simulink model "V30x2810x29"  (R2024b)
settings: Solver=ode1  StartTime=0.0  StopTime=inf  FixedStep=0.01  RelTol=1e-3  EnableMultiTasking=on
PostLoadFcn:
  | qlabs_setup
model workspace (MAT data in the model file):
  Sig = Simulink.Signal
  Sig.Dimensions = -1
  Sig.DimensionsMode = 'auto'
  Sig.Complexity = 'auto'
  Sig.SampleTime = -1
  Sig.SamplingMode = 'auto'
  Sig.DataType = 'auto'
  downCamStepSize = Simulink.Parameter
  downCamStepSize.Value = Simulink.data.Expression
  downCamStepSize.Value.ExpressionString = "qc_get_step_size*ceil(1/30/qc_get_step_size)"
  downCamStepSize.Complexity = 'real'
  downCamStepSize.Dimensions = -1
  downCamStepSize.DataType = 'auto'
  lidarStepSize = Simulink.Parameter
  lidarStepSize.Value = Simulink.data.Expression
  lidarStepSize.Value.ExpressionString = "qc_get_step_size*ceil(1/5/qc_get_step_size)"
  lidarStepSize.Complexity = 'real'
  lidarStepSize.Dimensions = -1
  lidarStepSize.DataType = 'auto'
  mainStepSize = Simulink.Parameter
  mainStepSize.Value = Simulink.data.Expression
  mainStepSize.Value.ExpressionString = "qc_get_step_size"
  mainStepSize.Complexity = 'real'
  mainStepSize.Dimensions = -1
  mainStepSize.DataType = 'auto'
  mode = Simulink.Parameter
  mode.Value = 2
  mode.Complexity = 'real'
  mode.Dimensions = [1 1]
  mode.Description = '0 - education speeds via wheel speed commands
    | 1 - education speeds via body speed commands
    | 2 - research speeds via wheel speed commands
    | 3 - research speeds via body speed commands'
  mode.DataType = 'auto'
  realSenseStepSize = Simulink.Parameter
  realSenseStepSize.Value = Simulink.data.Expression
  realSenseStepSize.Value.ExpressionString = "qc_get_step_size*ceil(1/30/qc_get_step_size)"
  realSenseStepSize.Complexity = 'real'
  realSenseStepSize.Dimensions = -1
  realSenseStepSize.DataType = 'auto'
values from neighbouring files (symbols this model uses):
  obstacles = [ ... (first row only)    [init.m]
  waypoints = [ ... (first row only)    [init.m]
libraries: quarc_library x7
settings Model: ExtModeTrigDuration=10000  Creator=mbohra  LastModifiedBy=simon
settings SolverCC: PositivePriorityOrder=on
settings DebuggingCC: UnderspecifiedInitializationDetection=Classic  MergeDetectMultiDrivingBlocksExec=none
settings ModelReferenceCC: PropagateSignalLabelsOutOfModel=off
settings RTWCC: Description=QUARC Win64 Target Using Toolchain  SystemTargetFile=quarc_win64.tlc  Toolchain=QUARC win64 | nmake (64-bit Windows)  BuildConfiguration=Faster Runs  GPUComputeCapability=3.5
settings STFCustomTargetCC: TargetLangStandard=C99 (ISO)  ConcurrentExecutionCompliant=on  GRTInterface=on  UseToolchainInfoCompliant=on  SystemTargetFile=quarc_win64.tlc
settings GRTTargetCC: ParMdlRefBuildCompliant=off  CompOptLevelCompliant=off  CombineOutputUpdateFcns=off  MatFileLogging=off  CPPClassGenCompliant=off  GRTInterface=on  ExtMode=on  ExtModeMexFile=quarc_comm

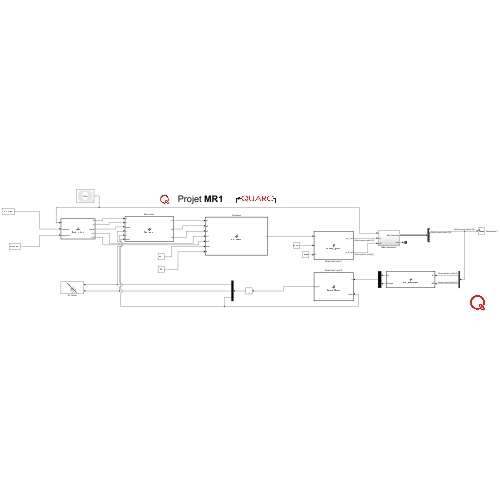
[thumbnail: Simulink's stored preview of the top-level diagram]
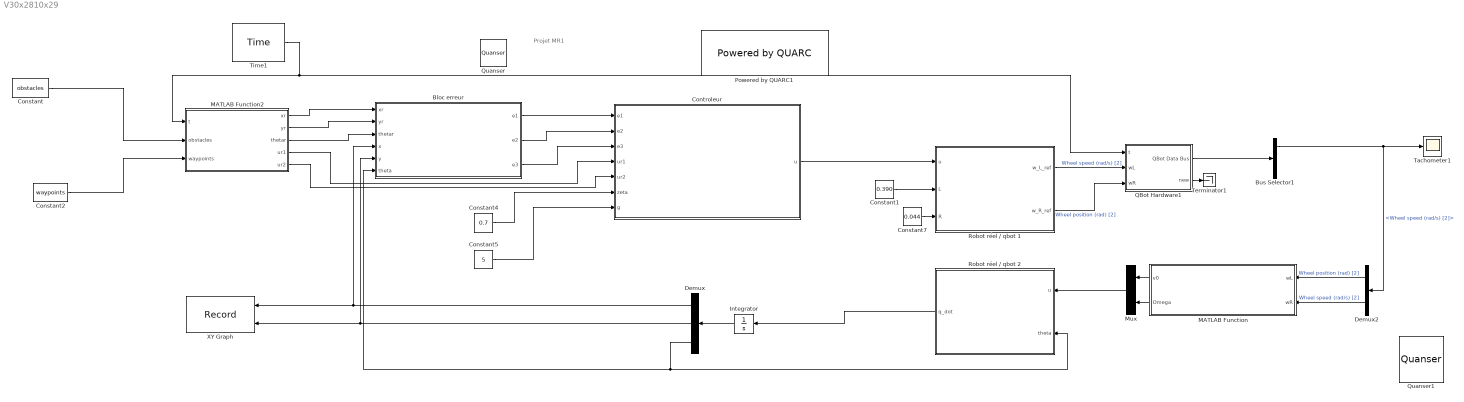
== system V30x2810x29 ==
  note: Projet MR1
  Bloc erreur : MATLAB Function  TreatAsAtomicUnit=on
  Bus Selector1 : BusSelector  OutputSignals=Wheel position (rad) [2],Wheel speed (rad/s) [2],Motor Cmd (Volts) [2],Acceleration (m/s/s) [3],Gyroscope (rad/s) [3],Current (Amps) [2],Battery (Volts)
  Constant : Constant  Value=obstacles
  Constant1 : Constant  Value=0.390
  Constant2 : Constant  Value=waypoints
  Constant4 : Constant  Value=0.7
  Constant5 : Constant  Value=5
  Constant7 : Constant  Value=0.044
  Controleur : MATLAB Function  TreatAsAtomicUnit=on
  Demux : Demux  Outputs=3
  Demux2 : Demux  Outputs=2
  Integrator : Integrator
  MATLAB Function : MATLAB Function  TreatAsAtomicUnit=on
  MATLAB Function2 : MATLAB Function  TreatAsAtomicUnit=on
  Mux : Mux  Inputs=2
  Powered by QUARC1 : quarc_library/Logos/Powered by QUARC
  QBot Hardware1 : Subsystem
  Quanser : quarc_library/Logos/Quanser
  Quanser1 : quarc_library/Logos/Quanser
  Robot réel / qbot 1 : MATLAB Function  TreatAsAtomicUnit=on
  Robot réel / qbot 2 : MATLAB Function  TreatAsAtomicUnit=on
  Tachometer1 : Scope
  Terminator1 : Terminator
  Time1 : quarc_library/Sources/Time/Time  time_source=Wall clock  sample_time=qc_get_step_size
  XY Graph : Record  FileSettingsInternal="{\"entries\":[{\"content\":{\"excelSettings\":{\"content\":{},\"type\":\"Streamout.ExcelSettings\"}},\"type\":\"Streamout.FileSettingStorage\",\"uuid\":\"\"}],\"packageUris\":[\"http:\\/\\/schema.mathworks.com\\/mf0\\/streamout_blocks\\/R2020a\"],\"version\":\"1.0\"}"  Layout=[1 1]  SignalsInternal="{\"entries\":[{\"content\":{\"signals\":[{\"content\":{\"blockPath\":[],\"dimensions\":[1,1],\"domain\":\"\",\"lineColor\":\"#a2142f\",\"plots\":[ 1 ],\"port\":1,\"sid\":[\"\"],\"signalID\":1,\"signalName\":\"Demux:1\"},\"type\":\"RecordBlkView.Signal\",\"uuid\":\"\"},{\"content\":{\"blockPath\":[],\"dimensions\":[1,1],\"domain\":\"\",\"lineColor\":\"#139fff\",\"plots\":[ 1 ],\"port\":2,\"sid\":[\"\"],\"signalID\":2,\"signalName\":\"Demux:2\"},\"type\":\"RecordBlkView.Signal\",\"uuid\":\"\"}]},\"type\":\"RecordBlkView.InputSignals\",\"uuid\":\"\"}],\"packageUris\":[\"http:\\/\\/schema.mathworks.com\\/mf0\\/streamout_blocks\\/R2020a\"],\"version\":\"1.0\"}"  VisualizationBindings="{\"xyplotplugin\":{\"info\":[{\"series\":[{\"bindingParametersList\":[{\"parameter\":\"X-Axis\",\"signalID\":1,\"signalName\":\"Demux:1\"},{\"parameter\":\"Y-Axis\",\"signalID\":2,\"signalName\":\"Demux:2\"}],\"seriesID\":0}],\"subplotID\":1}]}}"  CompatibilityTag=XY
  wires:
  Controleur/1(u) -> Robot réel / qbot 1/1(u)
  Constant4/1 -> Controleur/6(zeta)
  Demux/3 -> Robot réel / qbot 2/2(theta), Bloc erreur/6(theta)
  Robot réel / qbot 2/1(q_dot) -> Integrator/1
  Bloc erreur/1(e1) -> Controleur/1(e1)
  Demux2/1 -> MATLAB Function/1(wL)  "Wheel position (rad) [2]"
  Demux2/2 -> MATLAB Function/2(wR)  "Wheel speed (rad/s) [2]"
  MATLAB Function/2(Omega) -> Mux/2
  Constant1/1 -> Robot réel / qbot 1/2(L)
  Robot réel / qbot 1/1(w_L_ref) -> QBot Hardware1/2(wL)  "Wheel speed (rad/s) [2]"
  Constant5/1 -> Controleur/7(g)
  MATLAB Function2/4(ur1) -> Controleur/4(ur1)
  Time1/1 -> MATLAB Function2/1(t), QBot Hardware1/1(t)
  MATLAB Function/1(v0) -> Mux/1
  QBot Hardware1/2(new) -> Terminator1/1
  Bus Selector1/2 -> Demux2/1, Tachometer1/1  "<Wheel speed (rad/s) [2]>"
  MATLAB Function2/1(xr) -> Bloc erreur/1(xr)
  MATLAB Function2/5(ur2) -> Controleur/5(ur2)
  Integrator/1 -> Demux/1
  Bloc erreur/2(e2) -> Controleur/2(e2)
  Bloc erreur/3(e3) -> Controleur/3(e3)
  Demux/1 -> Bloc erreur/4(x), XY Graph/1
  QBot Hardware1/1(QBot Data Bus) -> Bus Selector1/1
  Robot réel / qbot 1/2(w_R_ref) -> QBot Hardware1/3(wR)  "Wheel position (rad) [2]"
  Constant7/1 -> Robot réel / qbot 1/3(R)
  MATLAB Function2/2(yr) -> Bloc erreur/2(yr)
  MATLAB Function2/3(thetar) -> Bloc erreur/3(thetar)
  Mux/1 -> Robot réel / qbot 2/1(u)
  Constant/1 -> MATLAB Function2/2(obstacles)
  Constant2/1 -> MATLAB Function2/3(waypoints)
  Demux/2 -> Bloc erreur/5(y), XY Graph/2

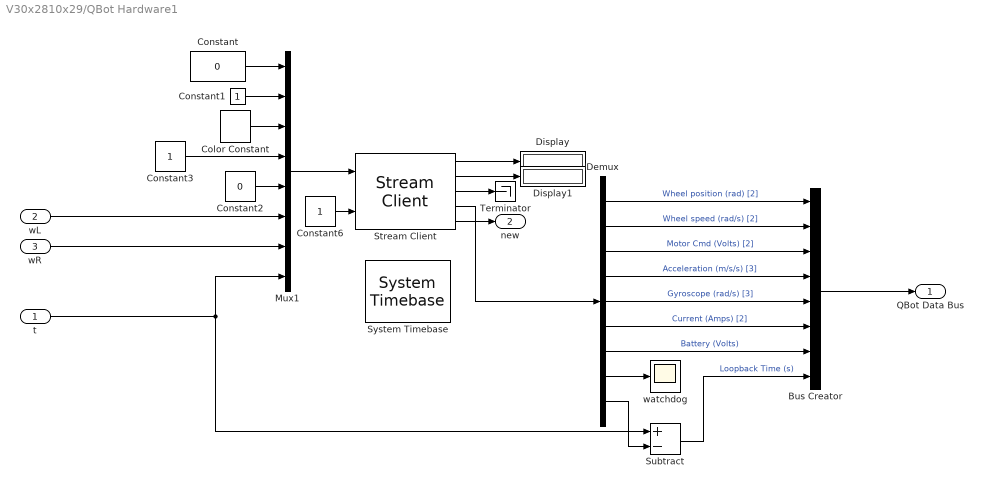
== system V30x2810x29/QBot Hardware1 ==
  t : Inport
  wL : Inport  Port=2
  wR : Inport  Port=3
  Bus Creator : BusCreator  Inputs=8
  Color Constant : quarc_library/Sources/Signals/Color Constant  color=[1 0.07451 0.65098]
      settings: SourceProductName=QUARC Targets
  Constant : Constant  Value=0
  Constant1 : Constant
  Constant2 : Constant  Value=0
  Constant3 : Constant
  Constant6 : Constant
  Demux : Demux  Outputs=[2 2 2 3 3 2 1 1 1]
  Display : Display
  Display1 : Display
  Mux1 : Mux  Inputs=8
  Stream Client : quarc_library/Communications/Basic/Stream Client  uri_source=Specify via dialog (do not evaluate)  uri=tcpip://localhost:18888  send_buffer_size=1460  receive_buffer_size=1460  byte_order=little endian (Intel - LSB first)  optimization=Minimum latency  send_options=Send most recent data  receive_options=Receive most recent data  default_value=zeros(17,1)  sample_time=qc_get_step_size  active=on  implementation=Use blocking I/O in a separate thread  send_fifo_size=1000  receive_fifo_size=1000  send_priority=0  receive_priority=0  send_dimensions=off  receive_dimensions=off  max_dimensions=-1  data_type=Inherited via back propagation  type_expr=BusObject
      settings: AttributesFormatString="\"tcpip://localhost:18888\""
  Subtract : Sum  Inputs=+-
  System Timebase : quarc_library/Advanced/Timing/System Timebase  stop_on_overrun=off
      settings: SourceProductName=QUARC Targets
  Terminator : Terminator
  watchdog : Scope
  QBot Data Bus : Outport
  new : Outport  Port=2
  wires:
  Demux/2 -> Bus Creator/2  "Wheel speed (rad/s) [2]"
  Constant/1 -> Mux1/1
  Stream Client/3 -> Terminator/1
  Stream Client/1 -> Display/1
  Constant6/1 -> Stream Client/2
  Stream Client/2 -> Display1/1
  Color Constant/1 -> Mux1/3
  Constant1/1 -> Mux1/2
  Demux/3 -> Bus Creator/3  "Motor Cmd (Volts) [2]"
  Mux1/1 -> Stream Client/1
  Stream Client/4 -> Demux/1
  Demux/1 -> Bus Creator/1  "Wheel position (rad) [2]"
  Stream Client/5 -> new/1
  Demux/7 -> Bus Creator/7  "Battery (Volts)"
  Demux/5 -> Bus Creator/5  "Gyroscope (rad/s) [3]"
  Demux/6 -> Bus Creator/6  "Current (Amps) [2]"
  Demux/9 -> Subtract/2
  Constant2/1 -> Mux1/5
  Demux/4 -> Bus Creator/4  "Acceleration (m/s/s) [3]"
  t/1 -> Subtract/1, Mux1/8
  Bus Creator/1 -> QBot Data Bus/1
  Subtract/1 -> Bus Creator/8  "Loopback Time (s)"
  Demux/8 -> watchdog/1
  Constant3/1 -> Mux1/4
  wL/1 -> Mux1/6
  wR/1 -> Mux1/7

== matlab function V30x2810x29/MATLAB Function2 ==
  data: t input; xr output; yr output; thetar output; ur1 output; ur2 output; obstacles input; waypoints input
function [xr, yr, thetar, ur1, ur2] = Traj_bezier3(t, obstacles, waypoints)
    % Entrée : t (temps de simulation)
    % Sorties : Références x, y, theta, v, omega

    coder.extrinsic('plot');

    % Mémoire pour stocker la trajectoire calculée une seule fois
    persistent time_ref x_ref y_ref theta_ref v_ref omega_ref initialized
    
    if isempty(initialized)
        v_max = 0.5;           
        omega_max = 2.0;       
                
        % Obstacles Rectangulaires [x, y, w, h, theta]
        obstacles_rect = [
            %1.0, 1.0, 2.0, 1, 0;    
        ];

        gates = [];
        n_points_per_seg = 1000; % Points par segment
        marge_securite = 0.5;

        % Initialisation des vecteurs totaux
        x_total = []; y_total = []; theta_total = [];
        v_total = []; omega_total = []; time_total = [];
        
        cumul_time = 0;
        
        % Boucle sur chaque segment (entre waypoint i et i+1)
        for seg = 1:(size(waypoints, 1) - 1)
            
            x_start = waypoints(seg, 1); y_start = waypoints(seg, 2); theta_start = waypoints(seg, 3);
            x_goal = waypoints(seg+1, 1); y_goal = waypoints(seg+1, 2); theta_goal = waypoints(seg+1, 3);
            
            % Tangentes -> points intermédiaires
            distance = sqrt((x_goal - x_start)^2 + (y_goal - y_start)^2);
            longueur_tangente = distance / 3;
             
            P0 = [x_start, y_start];
            P1 = P0 + longueur_tangente * [cos(theta_start), sin(theta_start)];
            P2 = [x_goal, y_goal] - longueur_tangente * [cos(theta_goal), sin(theta_goal)];
            P3 = [x_goal, y_goal];
            
            % On modifie les points intermédiaires s'ils sont trop proche
            % d'un obstacle
            for i = 1:size(obstacles, 1)
                obs_c = obstacles(i, 1:2); r_obs = obstacles(i, 3);
                
                % P1
                if norm(P1 - obs_c) < r_obs + marge_securite + 0.5
                    dir = (P1 - obs_c) / norm(P1 - obs_c);
                    P1 = obs_c + dir * (r_obs + marge_securite + 0.8);
                end
                % P2
                if norm(P2 - obs_c) < r_obs + marge_securite + 0.5
                    dir = (P2 - obs_c) / norm(P2 - obs_c);
                    P2 = obs_c + dir * (r_obs + marge_securite + 0.8);
                end
            end
            
            for i = 1:size(obstacles_rect, 1)
                xc = obstacles_rect(i, 1); yc = obstacles_rect(i, 2);
                W = obstacles_rect(i, 3); H = obstacles_rect(i, 4); ang = obstacles_rect(i, 5);
                R_mat = [cos(ang), -sin(ang); sin(ang), cos(ang)];
                corners_loc = [-W/2, -H/2; W/2, -H/2; W/2, H/2; -W/2, H/2];
                corners_glob = (R_mat * corners_loc')' + [xc, yc];
                r_coin = 0.3;
                
                % Vérifier P1 et P2 contre les 4 coins
                for j=1:4
                    coin = corners_glob(j,:);
                    if norm(P1 - coin) < r_coin + marge_securite + 0.5
                         dir = (P1 - coin)/norm(P1 - coin);
                         P1 = coin + dir * (r_coin + marge_securite + 0.8);
                    end
                    if norm(P2 - coin) < r_coin + marge_securite + 0.5
                         dir = (P2 - coin)/norm(P2 - coin);
                         P2 = coin + dir * (r_coin + marge_securite + 0.8);
                    end
                end
            end
            
            % génération de la trajectoire via Bezier
            tt = linspace(0, 1, n_points_per_seg)';
            x_seg = (1-tt).^3*P0(1) + 3*(1-tt).^2.*tt*P1(1) + 3*(1-tt).*tt.^2*P2(1) + tt.^3*P3(1);
            y_seg = (1-tt).^3*P0(2) + 3*(1-tt).^2.*tt*P1(2) + 3*(1-tt).*tt.^2*P2(2) + tt.^3*P3(2);
            

            dx = gradient(x_seg); dy = gradient(y_seg);
            theta_seg = atan2(dy, dx);
            
            ddx = gradient(dx); ddy = gradient(dy);
            kappa = (dx.*ddy - dy.*ddx) ./ (dx.^2 + dy.^2).^(3/2);
            kappa(isnan(kappa)) = 0;
            
            % Profil de vitesse
            v_seg = v_max * ones(size(kappa));
            for k=1:length(kappa)
                if abs(kappa(k)) > 0.01 % si la courbure est trop elevee on ralentit
                    v_lim = sqrt(3.0 / abs(kappa(k)));
                    v_seg(k) = min(v_seg(k), v_lim);
                end
            end
            v_seg = min(v_seg, v_max);
            
            omega_seg = v_seg .* kappa;
            omega_seg = max(min(omega_seg, omega_max), -omega_max);
            
            % conversion du temps de bezier ([0,1]) en un temps reel base
            % sur le calcul du temp total
            ds = sqrt(diff(x_seg).^2 + diff(y_seg).^2);
            ds = [0; ds];
            dt = ds ./ max(v_seg, 0.01);
            time_seg = cumsum(dt) + cumul_time;

            if seg == 1
                x_total = [x_total; x_seg];
                y_total = [y_total; y_seg];
                theta_total = [theta_total; theta_seg];
                v_total = [v_total; v_seg];
                omega_total = [omega_total; omega_seg];
                time_total = [time_total; time_seg];
            else
                % On saute le premier point pour éviter les doublons
                x_total = [x_total; x_seg(2:end)];
                y_total = [y_total; y_seg(2:end)];
                theta_total = [theta_total; theta_seg(2:end)];
                v_total = [v_total; v_seg(2:end)];
                omega_total = [omega_total; omega_seg(2:end)];
                time_total = [time_total; time_seg(2:end)];
            end
            
            cumul_time = time_total(end);
        end
        
        % Correction finale des angles (Unwrap) pour éviter les sauts +/- Pi
        theta_total = unwrap(theta_total);

        % Stockage Persistant
        time_ref = time_total;
        x_ref = x_total;
        y_ref = y_total;
        theta_ref = theta_total;
        v_ref = v_total;
        omega_ref = omega_total;

        figure('Name', 'Trajectoire Bézier Multi-Points', 'Position', [970 100 900 700]);
        hold on; grid on; axis equal;
        
        % Dessiner obstacles circulaires
        for i = 1:size(obstacles, 1)
            circle_x = obstacles(i,1) + obstacles(i,3) * cos(0:0.01:2*pi);
            circle_y = obstacles(i,2) + obstacles(i,3) * sin(0:0.01:2*pi);
            fill(circle_x, circle_y, [1 0.7 0.7], 'EdgeColor', 'r', 'LineWidth', 2);
        end

        % Dessiner la trajectoire complète
        plot(x_ref, y_ref, 'b-', 'LineWidth', 3);
        
        % Dessiner les waypoints
        for i = 1:size(waypoints, 1)
            if i == 1
                % Point de départ (vert)
                plot(waypoints(i,1), waypoints(i,2), 'go', 'MarkerSize', 15, 'MarkerFaceColor', 'g');
                quiver(waypoints(i,1), waypoints(i,2), 0.4*cos(waypoints(i,3)), ...
                       0.4*sin(waypoints(i,3)), 0, 'g', 'LineWidth', 3, 'MaxHeadSize', 1);
            elseif i == size(waypoints, 1)
                % Point d'arrivée final (rouge)
                plot(waypoints(i,1), waypoints(i,2), 'ro', 'MarkerSize', 15, 'MarkerFaceColor', 'r');
                quiver(waypoints(i,1), waypoints(i,2), 0.4*cos(waypoints(i,3)), ...
                       0.4*sin(waypoints(i,3)), 0, 'r', 'LineWidth', 3, 'MaxHeadSize', 1);
            else
                % Points intermédiaires (bleu)
                plot(waypoints(i,1), waypoints(i,2), 'bo', 'MarkerSize', 12, 'MarkerFaceColor', 'b');
                quiver(waypoints(i,1), waypoints(i,2), 0.4*cos(waypoints(i,3)), ...
                       0.4*sin(waypoints(i,3)), 0, 'b', 'LineWidth', 2, 'MaxHeadSize', 1);
            end
        end
        
        initialized = 1;
    end
    
    
    if t > time_ref(end)
        % Fin de la trajectoire : on reste sur place
        xr = x_ref(end);
        yr = y_ref(end);
        thetar = theta_ref(end);
        ur1 = 0; % Vitesse linéaire nulle
        ur2 = 0; % Vitesse angulaire nulle
    else
        % on trouve les valeurs exactes au temp t en interpolant dans les
        % tableaux calcule
        % Interpolation
        xr = interp1(time_ref, x_ref, t, 'spline');
        yr = interp1(time_ref, y_ref, t, 'spline');
        thetar = interp1(time_ref, theta_ref, t, 'spline');
        ur1 = interp1(time_ref, v_ref, t, 'spline');
        ur2 = interp1(time_ref, omega_ref, t, 'spline');
    end
    xfull = x_ref;
    yfull = y_ref;
end

== matlab function V30x2810x29/Bloc erreur ==
  data: e1 output; xr input; yr input; thetar input; x input; y input; theta input; e2 output; e3 output
function [e1, e2, e3] = Bloc_erreur(xr, yr, thetar, x, y, theta)

    % Calcul des erreurs dans le repère global
    ex_global = xr - x;
    ey_global = yr - y;
    etheta_global = thetar - theta;


    % Normalisation de l'angle de -pi à pi
    etheta_global = atan2(sin(etheta_global), cos(etheta_global));

    % Matrice de Rotattion de l'équation 5 du paper
    e1 =  cos(theta) * ex_global + sin(theta) * ey_global;
    e2 = -sin(theta) * ex_global + cos(theta) * ey_global;
    e3 = etheta_global;

    
end

== matlab function V30x2810x29/Controleur ==
  data: e1 input; e2 input; e3 input; u output; ur1 input; ur2 input; zeta input; g input
function u = Controlleur(e1, e2, e3, ur1, ur2, zeta, g)

    % Gain Scheduling + équation 1_ et 19

        wn = sqrt(ur2^2 + g*ur1^2);

        % Calcul des gains
        k1 = 2*zeta*wn;
        k3 = k1;                        % dans l'équation 15, k1 = k3
        k2 = g*abs(ur1);                % gain variable selon la vitesse
    
    % Calcul des corrections feedback -> équatioon 11
        v1 = -k1 * e1;
        v2 = -sign(ur1)*k2*e2 - k3*e3;
        % v1 = 0;
        % v2 = 0;

    % Commande totaleuuuu Feedforward + Feedback -> équation 7
        u1 = ur1 *cos(e3) - v1;
        u2 = ur2 - v2;
        

        u = [u1; u2];
end

== matlab function V30x2810x29/MATLAB Function ==
  data: wL input; v0 output; wR input; Omega output
function [v0, Omega] = Fwd_Kinematics(wL, wR)
    % wL : Vitesse angulaire roue gauche (rad/s)
    % wR : Vitesse angulaire roue droite (rad/s)
    % R  : Rayon de la roue (m)
    % L  : Entraxe (distance entre les roues en m)

    R = 0.044;   % Rayon de la roue (44 mm)
    L = 0.390;   % Entraxe entre les roues (39 cm)

    % 1. Conversion en vitesse linéaire de chaque roue (m/s)
    v_left = wL * R;
    v_right = wR * R;

    % 2. Calcul de la vitesse linéaire du robot (v0)
    % C'est la moyenne des deux roues
    v0 = (v_right + v_left) / 2;

    % 3. Calcul de la vitesse de rotation du robot (Omega)
    % C'est la différence de vitesse divisée par la largeur du robot
    Omega = (v_right - v_left) / L;
    
end

== matlab function V30x2810x29/Robot réel // qbot 1 ==
  data: w_L_ref output; u input; w_R_ref output; L input; R input
function [w_L_ref, w_R_ref] = Motors_Speed(u, L, R)
    % u(1) = u1 (Vitesse linéaire v en m/s)
    % u(2) = u2 (Vitesse angulaire omega en rad/s)

    v = u(1);
    omega = u(2);

    % Calcul des vitesses linéaires de chaque roue 
    w_L_ref = (2*v-L*omega)/(2*R);
    w_R_ref = (2*v+L*omega)/(2*R);
    % Conversion en vitesse angulaire (rad/s) pour les moteurs
    %w_R_ref = (v_R / R);
    %w_L_ref = (v_L / R);
end

== matlab function V30x2810x29/Robot réel // qbot 2 ==
  data: u input; q_dot output; theta input
function q_dot  = Robot_Model(u, theta)
    % u(1) = u1 (vitesse linéaire)
    % u(2) = u2 (vitesse angulaire)

    q_dot = [0;0;0];
    q_dot(1) = u(1) * cos(theta);
    q_dot(2) = u(1) * sin(theta);
    q_dot(3) = u(2);
end
